simulink model "problem5"  (R2020b)
settings: Solver=VariableStepAuto  StartTime=0.0  StopTime=10.0  MaxStep=.001  RelTol=1e-3
values from neighbouring files (symbols this model uses):
  c = 10/1000000    (= 1e-05)    [problem5data.m]
  r = 10    [problem5data.m]
settings Model: Creator=SAGAR  LastModifiedBy=SAGAR
settings DataIOCC: ExternalInput=[t,u]  SaveFormat=Array

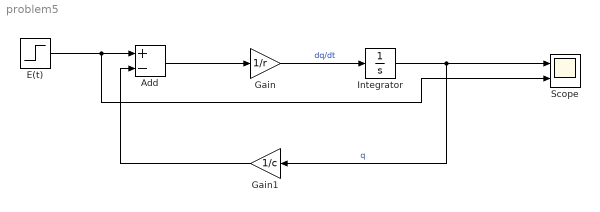
== system problem5 ==
  Add : Sum  Inputs=+-
  E(t) : Step  After=5  SampleTime=0
  Gain : Gain  Gain=1/r
  Gain1 : Gain  Gain=1/c
  Integrator : Integrator  InitialCondition=1
  Scope : Scope  NumInputPorts=2
  wires:
  E(t)/1 -> Scope/2, Add/1
  Add/1 -> Gain/1
  Gain/1 -> Integrator/1  "dq/dt"
  Integrator/1 -> Scope/1, Gain1/1  "q"
  Gain1/1 -> Add/2
